simulink model "gm_reverb_fdn"  (R2024a)
settings: Solver=FixedStepAuto  StartTime=0.0  StopTime=8  RelTol=1e-3
settings Model: Creator=fermata  LastModifiedBy=fermata
settings OptimizationCC: BlockReduction=off  ConditionallyExecuteInputs=off
settings DebuggingCC: InheritedTsInSrcMsg=none

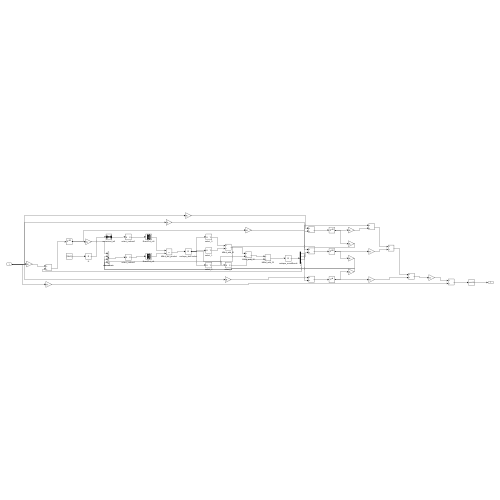
[thumbnail: Simulink's stored preview of the top-level diagram]
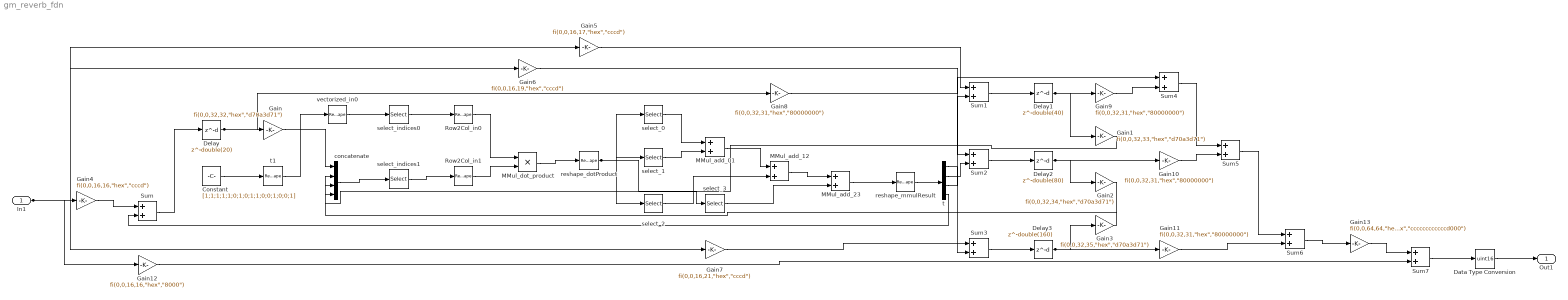
== system gm_reverb_fdn ==
  In1 : Inport  OutDataTypeStr=uint16  PortDimensions=1  SampleTime=0.16
  Constant : Constant  Value=[1;1;1;1;1;0;1;0;1;1;0;0;1;0;0;1]  OutDataTypeStr=uint16  SampleTime=0.16
  Data Type Conversion : DataTypeConversion  OutDataTypeStr=uint16  SampleTime=0.16  SaturateOnIntegerOverflow=off  RndMeth=Floor
  Delay : Delay  DelayLength=double(20)  InitialCondition=0  SampleTime=0.16
  Delay1 : Delay  DelayLength=double(40)  InitialCondition=0  SampleTime=0.16
  Delay2 : Delay  DelayLength=double(80)  InitialCondition=0  SampleTime=0.16
  Delay3 : Delay  DelayLength=double(160)  InitialCondition=0  SampleTime=0.16
  Gain : Gain  Gain="fi(0,0,32,32,\"hex\",\"d70a3d71\")"  ParamDataTypeStr=fixdt(0, 32, 32)  OutDataTypeStr=uint16  RndMeth=Simplest  SaturateOnIntegerOverflow=on  SampleTime=0.16
  Gain1 : Gain  Gain="fi(0,0,32,33,\"hex\",\"d70a3d71\")"  ParamDataTypeStr=fixdt(0, 32, 33)  OutDataTypeStr=uint16  RndMeth=Simplest  SaturateOnIntegerOverflow=on  SampleTime=0.16
  Gain{8..11} (4 alike) : Gain  Gain="fi(0,0,32,31,\"hex\",\"80000000\")"  ParamDataTypeStr=fixdt(0, 32, 31)  OutDataTypeStr=fixdt(0, 64, 31)  SampleTime=0.16
  Gain12 : Gain  Gain="fi(0,0,16,16,\"hex\",\"8000\")"  ParamDataTypeStr=fixdt(0, 16, 16)  OutDataTypeStr=fixdt(0, 32, 16)  SampleTime=0.16
  Gain13 : Gain  Gain="fi(0,0,64,64,\"hex\",\"ccccccccccccd000\")"  ParamDataTypeStr=fixdt(0, 64, 64)  OutDataTypeStr=fixdt(0, 128, 95)  SampleTime=0.16
  Gain2 : Gain  Gain="fi(0,0,32,34,\"hex\",\"d70a3d71\")"  ParamDataTypeStr=fixdt(0, 32, 34)  OutDataTypeStr=uint16  RndMeth=Simplest  SaturateOnIntegerOverflow=on  SampleTime=0.16
  Gain3 : Gain  Gain="fi(0,0,32,35,\"hex\",\"d70a3d71\")"  ParamDataTypeStr=fixdt(0, 32, 35)  OutDataTypeStr=uint16  RndMeth=Simplest  SaturateOnIntegerOverflow=on  SampleTime=0.16
  Gain4 : Gain  Gain="fi(0,0,16,16,\"hex\",\"cccd\")"  ParamDataTypeStr=fixdt(0, 16, 16)  OutDataTypeStr=fixdt(0, 32, 16)  SampleTime=0.16
  Gain5 : Gain  Gain="fi(0,0,16,17,\"hex\",\"cccd\")"  ParamDataTypeStr=fixdt(0, 16, 17)  OutDataTypeStr=fixdt(0, 32, 17)  SampleTime=0.16
  Gain6 : Gain  Gain="fi(0,0,16,19,\"hex\",\"cccd\")"  ParamDataTypeStr=fixdt(0, 16, 19)  OutDataTypeStr=fixdt(0, 32, 19)  SampleTime=0.16
  Gain7 : Gain  Gain="fi(0,0,16,21,\"hex\",\"cccd\")"  ParamDataTypeStr=fixdt(0, 16, 21)  OutDataTypeStr=fixdt(0, 32, 21)  SampleTime=0.16
  MMul_add_01 : Sum  OutDataTypeStr=uint32  SaturateOnIntegerOverflow=on  SampleTime=0.16
  MMul_add_12 : Sum  OutDataTypeStr=uint32  SaturateOnIntegerOverflow=on  SampleTime=0.16
  MMul_add_23 : Sum  OutDataTypeStr=uint32  SaturateOnIntegerOverflow=on  SampleTime=0.16
  MMul_dot_product : Product  Inputs=**  OutDataTypeStr=uint32  SaturateOnIntegerOverflow=on  SampleTime=0.16
  Row2Col_in0 : Reshape  OutputDimensionality=Column vector (2-D)
  Row2Col_in1 : Reshape  OutputDimensionality=Column vector (2-D)
  Sum{,1..3} (4 alike) : Sum  OutDataTypeStr=uint32  AccumDataTypeStr=uint32  SampleTime=0.16
  Sum4 : Sum  OutDataTypeStr=fixdt(0, 64, 31)  AccumDataTypeStr=fixdt(0, 64, 31)  SampleTime=0.16
  Sum5 : Sum  OutDataTypeStr=fixdt(0, 64, 31)  AccumDataTypeStr=fixdt(0, 64, 31)  SampleTime=0.16
  Sum6 : Sum  OutDataTypeStr=fixdt(0, 64, 31)  AccumDataTypeStr=fixdt(0, 64, 31)  SampleTime=0.16
  Sum7 : Sum  OutDataTypeStr=fixdt(0, 128, 95)  AccumDataTypeStr=fixdt(0, 128, 95)  SampleTime=0.16
  concatenate : Concatenate  NumInputs=4  Mode=Multidimensional array  ConcatenateDimension=2
  reshape_dotProduct : Reshape  OutputDimensionality=Customize  OutputDimensions=[4,4]
  reshape_mmulResult : Reshape  OutputDimensionality=Customize  OutputDimensions=[4,1]
  select_0 : Selector  NumberOfDimensions=2  IndexOptions=Index vector (dialog),Select all  Indices=double(1),[]  OutputSizes=1
  select_1 : Selector  NumberOfDimensions=2  IndexOptions=Index vector (dialog),Select all  Indices=double(2),[]  OutputSizes=1
  select_2 : Selector  NumberOfDimensions=2  IndexOptions=Index vector (dialog),Select all  Indices=double(3),[]  OutputSizes=1
  select_3 : Selector  NumberOfDimensions=2  IndexOptions=Index vector (dialog),Select all  Indices=double(4),[]  OutputSizes=1
  select_indices0 : Selector  InputPortWidth=16  IndexOptions=Index vector (dialog)  Indices=double([1 5 9 13 2 6 10 14 3 7 11 15 4 8 12 16])  OutputSizes=1
  select_indices1 : Selector  InputPortWidth=4  IndexOptions=Index vector (dialog)  Indices=double([1 2 3 4 1 2 3 4 1 2 3 4 1 2 3 4])  OutputSizes=1
  t : Demux
  t1 : Reshape  OutputDimensionality=Customize  OutputDimensions=[4,4]
  vectorized_in0 : Reshape  OutputDimensionality=Row vector (2-D)
  Out1 : Outport  SampleTime=0.16
  wires:
  In1/1 -> Gain7/1, Gain6/1, Gain5/1, Gain4/1, Gain12/1
  t1/1 -> vectorized_in0/1
  Data Type Conversion/1 -> Out1/1
  Delay/1 -> Gain8/1, Gain/1
  Delay1/1 -> Gain9/1, Gain1/1
  Delay2/1 -> Gain2/1, Gain10/1
  Delay3/1 -> Gain3/1, Gain11/1
  Gain/1 -> concatenate/1
  Gain1/1 -> concatenate/2
  Gain10/1 -> Sum5/2
  Gain11/1 -> Sum6/2
  Gain12/1 -> Sum7/2
  Gain13/1 -> Sum7/1
  Gain2/1 -> concatenate/3
  Gain3/1 -> concatenate/4
  Gain4/1 -> Sum/1
  Gain5/1 -> Sum1/1
  Gain6/1 -> Sum2/1
  Gain7/1 -> Sum3/1
  Gain8/1 -> Sum4/1
  Gain9/1 -> Sum4/2
  concatenate/1 -> select_indices1/1
  reshape_mmulResult/1 -> t/1
  Sum/1 -> Delay/1
  Sum1/1 -> Delay1/1
  Sum2/1 -> Delay2/1
  Sum3/1 -> Delay3/1
  Sum4/1 -> Sum5/1
  Sum5/1 -> Sum6/1
  Sum6/1 -> Gain13/1
  Sum7/1 -> Data Type Conversion/1
  t/1 -> Sum3/2
  t/2 -> Sum2/2
  t/3 -> Sum1/2
  t/4 -> Sum/2
  Constant/1 -> t1/1
  vectorized_in0/1 -> select_indices0/1
  select_indices0/1 -> Row2Col_in0/1
  select_indices1/1 -> Row2Col_in1/1
  Row2Col_in0/1 -> MMul_dot_product/1
  Row2Col_in1/1 -> MMul_dot_product/2
  MMul_dot_product/1 -> reshape_dotProduct/1
  reshape_dotProduct/1 -> select_3/1, select_2/1, select_1/1, select_0/1
  select_0/1 -> MMul_add_01/1
  select_1/1 -> MMul_add_01/2
  MMul_add_01/1 -> MMul_add_12/1
  select_2/1 -> MMul_add_12/2
  MMul_add_12/1 -> MMul_add_23/1
  select_3/1 -> MMul_add_23/2
  MMul_add_23/1 -> reshape_mmulResult/1
